simulink model "lab3_dd_move"  (R2024b)
settings: Solver=FixedStepDiscrete  StartTime=0.0  StopTime=25  FixedStep=0.01  RelTol=1e-3
model workspace (MAT data in the model file):
  l = 0.1
  r = 0.05
libraries: mobileRoboticsTrainingLib x2, mobileRoboticsLib x1
settings Model: Creator=gtewolde  LastModifiedBy=Matthew
settings SolverCC: AlgebraicLoopSolver=TrustRegion
settings DebuggingCC: UnconnectedInputMsg=warning  UnconnectedOutputMsg=warning  UnconnectedLineMsg=warning
settings ModelReferenceCC: EnableRefExpFcnMdlSchedulingChecks=on
settings RTWCC: GPUComputeCapability=3.5

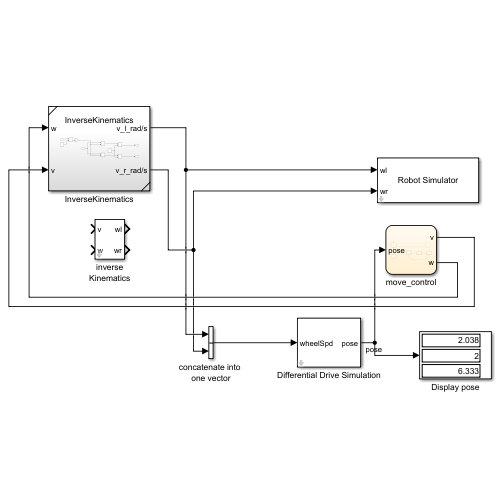
[thumbnail: Simulink's stored preview of the top-level diagram]
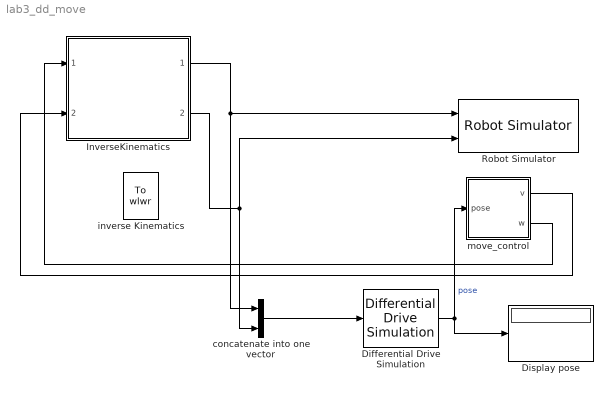
== system lab3_dd_move ==
  Differential Drive Simulation : mobileRoboticsLib/Kinematic Models/Differential Drive/Differential Drive Simulation  wheelRadius=0.05  wheelBase=0.1  initX=0.5  initY=0.5  initAngle=0  Ts=0.05
      settings: SourceProductName=Mobile Robotics Simulation Toolbox
  Display pose : Display
  InverseKinematics : Subsystem  ReferencedSubsystem=InverseKinematics
  Robot Simulator : mobileRoboticsTrainingLib/Robot Simulator  Priority=99  mapVar=[]  startX=0.5  startY=0.5  startTheta=0  axleLength=0.1  wheelR=0.05
  concatenate into one vector : Concatenate
  inverse Kinematics : mobileRoboticsTrainingLib/To wlwr  axleLength=0.1  wheelR=0.05
  move_control : Stateflow chart  TreatAsAtomicUnit=on
  wires:
  InverseKinematics/1 -> concatenate into one vector/1, Robot Simulator/1
  InverseKinematics/2 -> concatenate into one vector/2, Robot Simulator/2
  Differential Drive Simulation/1 -> move_control/1(pose), Display pose/1  "pose"
  move_control/1(v) -> InverseKinematics/2
  move_control/2(w) -> InverseKinematics/1
  concatenate into one vector/1 -> Differential Drive Simulation/1

== stateflow chart lab3_dd_move/move_control ==
  state Forward
    entry:
    v = 1;
    w = 0;
  state CCW
    entry:
    v = 0;
    w = 1;
    step = step + 1;
  state Circle
    entry:
    v=1;
    w=4/3;
  state Circle1
    entry:
    v=1;
    w=-4/3;
  state Circle2
    entry:
    v=1;
    w=-4/3;
  state Stop1
    entry:
    v = 0;
    w = 0;
  Forward -> CCW [order 1] : [(pose(1)>=3.5 && step == 0) || (pose(2)>=3.5 && step == 1) || (pose(1)<=0.5 && step == 2)]
  CCW -> Forward : [pose(3) >= (1.57079633 * (step))]
  Forward -> Stop1 [order 2] : [pose(2) <= 0.5 && step==3]
  (default) -> Circle
  Circle1 -> Circle2 : [pose(1)<=2]
  Circle -> Circle1 : [pose(3)>=2*pi]
  Circle2 -> Circle : [pose(1)>=2]
  data: pose input; v output; w output; step local =0
